simulink library "Brakes"  (R2024a)
settings: Solver=VariableStepAuto  StartTime=0.0  StopTime=10.0  RelTol=1e-3
undefined symbols (not defined in the file or in its folder): raptor_xcp_function
libraries: Raptor_lib x3, Utilities x2, simulink x1
settings Model: Creator=serga  LastModifiedBy=serga

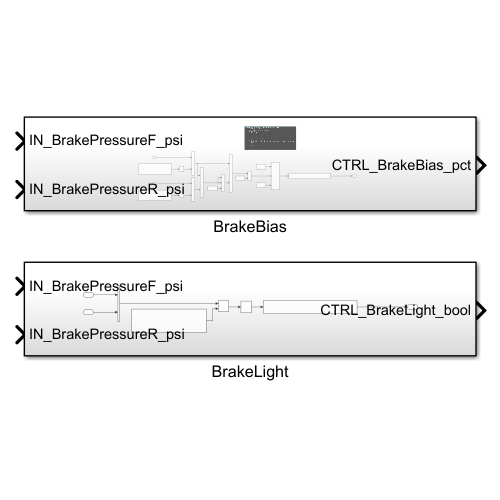
[thumbnail: Simulink's stored preview of the top-level diagram]
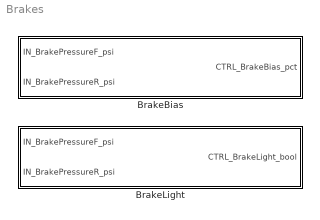
== system Brakes ==
  BrakeBias : Subsystem
  BrakeLight : Subsystem

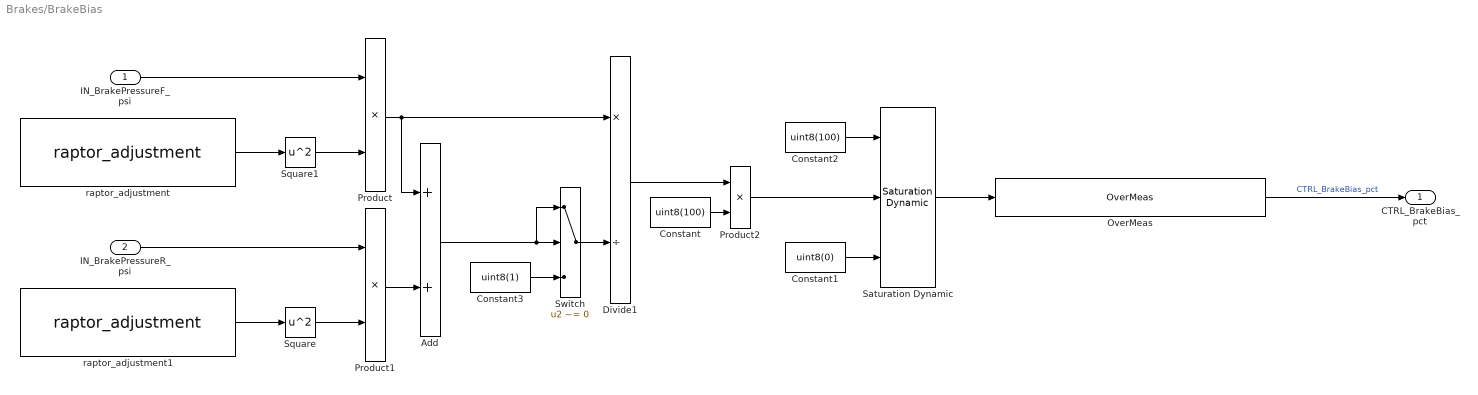
== system Brakes/BrakeBias ==
  IN_BrakePressureF_psi : Inport
  IN_BrakePressureR_psi : Inport  Port=2
  Add : Sum
  Constant : Constant  Value=uint8(100)
  Constant1 : Constant  Value=uint8(0)
  Constant2 : Constant  Value=uint8(100)
  Constant3 : Constant  Value=uint8(1)
  Divide1 : Product  Inputs=*/
  OverMeas : Utilities/OverMeas  sigName='CTRL_BrakeBias_pct'  minimum=0  maximum=100
  Product : Product
  Product1 : Product
  Product2 : Product
  Saturation Dynamic : simulink/Discontinuities/Saturation Dynamic  OutMin=[]  OutMax=[]  OutDataTypeStr=Inherit: Same as second input  OutDataType=fixdt(1, 16)  OutScaling=2^-10  DoSatur=off
  Square : Math  Operator=square
  Square1 : Math  Operator=square
  Switch : Switch  Criteria=u2 ~= 0  SaturateOnIntegerOverflow=off  InputSameDT=off
  raptor_adjustment : Raptor_lib/Data Storage/raptor_adjustment  paramName='CTRL_FrontPistonRadius_mm'  nameSource=Parameter  initValue=17  dataType=single  storage=Calibration  calDispType=Number  calEnum={'False', 'True'}  calGain=1.0  calOffset=0.0  calMax=50  calMin=0  calFormat='-1'  calUnit=''  calHelp=''  calAccess=1  calFunction=raptor_xcp_function(gcb)  calDispHeaders=off  calColHeaders={'Col1' 'Col2' 'Col3'}  calRowHeaders={'Row1' 'Row2' 'Row3'}
      settings: SourceProductName=Raptor
  raptor_adjustment1 : Raptor_lib/Data Storage/raptor_adjustment  paramName='CTRL_RearPistonRadius_mm'  nameSource=Parameter  initValue=12  dataType=single  storage=Calibration  calDispType=Number  calEnum={'False', 'True'}  calGain=1.0  calOffset=0.0  calMax=50  calMin=0  calFormat='-1'  calUnit=''  calHelp=''  calAccess=1  calFunction=raptor_xcp_function(gcb)  calDispHeaders=off  calColHeaders={'Col1' 'Col2' 'Col3'}  calRowHeaders={'Row1' 'Row2' 'Row3'}
      settings: SourceProductName=Raptor
  CTRL_BrakeBias_pct : Outport
  wires:
  OverMeas/1 -> CTRL_BrakeBias_pct/1  "CTRL_BrakeBias_pct"
  Saturation Dynamic/1 -> OverMeas/1
  Square/1 -> Product1/2
  Switch/1 -> Divide1/2
  Constant1/1 -> Saturation Dynamic/3
  Square1/1 -> Product/2
  Product1/1 -> Add/2
  Constant3/1 -> Switch/3
  raptor_adjustment/1 -> Square1/1
  Constant2/1 -> Saturation Dynamic/1
  Product/1 -> Divide1/1, Add/1
  Add/1 -> Switch/2, Switch/1
  Constant/1 -> Product2/2
  IN_BrakePressureR_psi/1 -> Product1/1
  Divide1/1 -> Product2/1
  IN_BrakePressureF_psi/1 -> Product/1
  Product2/1 -> Saturation Dynamic/2
  raptor_adjustment1/1 -> Square/1

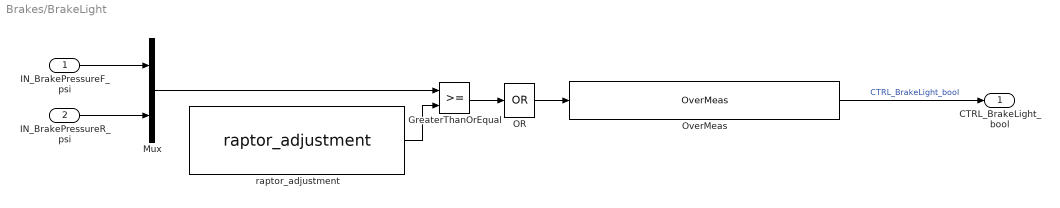
== system Brakes/BrakeLight ==
  IN_BrakePressureF_psi : Inport
  IN_BrakePressureR_psi : Inport  Port=2
  GreaterThanOrEqual : RelationalOperator  OutDataTypeStr=boolean  RndMeth=Simplest  InputSameDT=off
  Mux : Mux  Inputs=2
  OR : Logic  Operator=OR  Inputs=1  AllPortsSameDT=off  OutDataTypeStr=boolean
  OverMeas : Utilities/OverMeas  sigName='CTRL_BrakeLight_bool'  minimum=0  maximum=1
  raptor_adjustment : Raptor_lib/Data Storage/raptor_adjustment  paramName='CTRL_BrakeLightThresh_psi'  nameSource=Parameter  initValue=20  dataType=single  storage=Calibration  calDispType=Number  calEnum={'False', 'True'}  calGain=1.0  calOffset=0.0  calMax=2000  calMin=0  calFormat='-1'  calUnit=''  calHelp=''  calAccess=1  calFunction=raptor_xcp_function(gcb)  calDispHeaders=off  calColHeaders={'Col1' 'Col2' 'Col3'}  calRowHeaders={'Row1' 'Row2' 'Row3'}
      settings: SourceProductName=Raptor
  CTRL_BrakeLight_bool : Outport
  wires:
  OR/1 -> OverMeas/1
  IN_BrakePressureF_psi/1 -> Mux/1
  IN_BrakePressureR_psi/1 -> Mux/2
  Mux/1 -> GreaterThanOrEqual/1
  raptor_adjustment/1 -> GreaterThanOrEqual/2
  GreaterThanOrEqual/1 -> OR/1
  OverMeas/1 -> CTRL_BrakeLight_bool/1  "CTRL_BrakeLight_bool"
